simulink model "Blood_Platelet_Count_V2"  (R2022a)
settings: Solver=VariableStepAuto  StartTime=0.0  StopTime=10.0  RelTol=1e-3
model workspace (MAT data in the model file):
  Var = 0
settings Model: Creator=KVJ RAMAN  LastModifiedBy=KVJ RAMAN

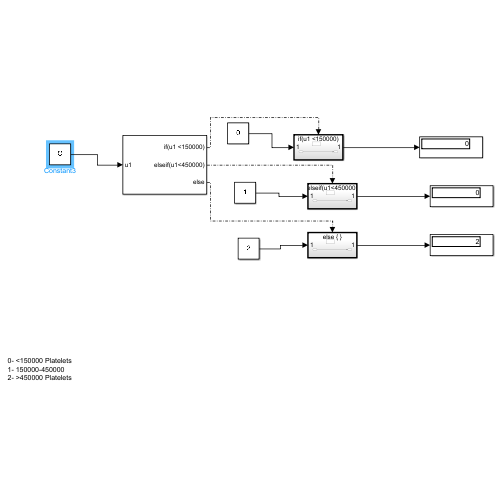
[thumbnail: Simulink's stored preview of the top-level diagram]
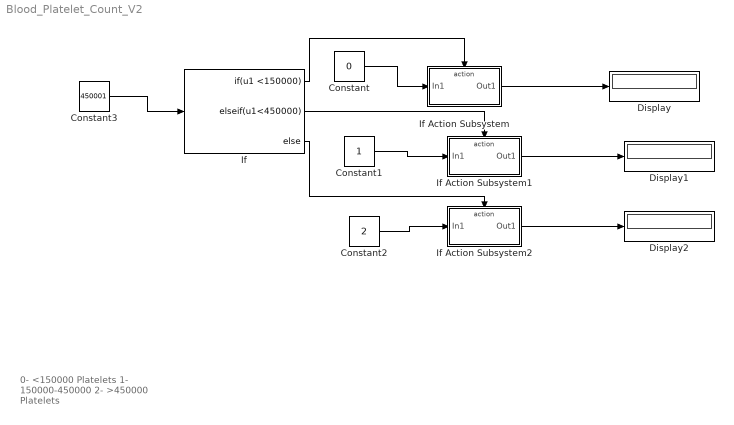
== system Blood_Platelet_Count_V2 ==
  note: 0- <150000 Platelets
      | 1- 150000-450000
      | 2- >450000 Platelets
  Constant : Constant  Value=0
  Constant1 : Constant
  Constant2 : Constant  Value=2
  Constant3 : Constant  Value=450001
  Display : Display
  Display1 : Display
  Display2 : Display
  If : If  IfExpression=u1 <150000  ElseIfExpressions=u1<450000
  If Action Subsystem : Subsystem  TreatAsAtomicUnit=on
  If Action Subsystem1 : Subsystem  TreatAsAtomicUnit=on
  If Action Subsystem2 : Subsystem  TreatAsAtomicUnit=on
  wires:
  If/1 -> If Action Subsystem/Action
  Constant/1 -> If Action Subsystem/1(In1)
  If/2 -> If Action Subsystem1/Action
  If/3 -> If Action Subsystem2/Action
  Constant1/1 -> If Action Subsystem1/1(In1)
  Constant2/1 -> If Action Subsystem2/1(In1)
  If Action Subsystem/1(Out1) -> Display/1
  If Action Subsystem1/1(Out1) -> Display1/1
  If Action Subsystem2/1(Out1) -> Display2/1
  Constant3/1 -> If/1

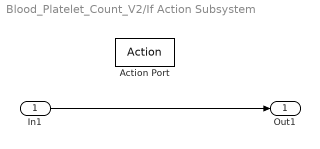
== system Blood_Platelet_Count_V2/If Action Subsystem ==
  In1 : Inport
  Action Port : ActionPort  ActionPortLabel=if(u1 <150000)
  Out1 : Outport
  wires:
  In1/1 -> Out1/1

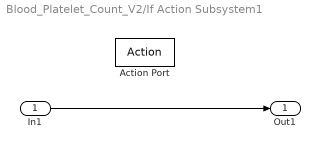
== system Blood_Platelet_Count_V2/If Action Subsystem1 ==
  In1 : Inport
  Action Port : ActionPort  ActionPortLabel=elseif(u1<450000)
  Out1 : Outport
  wires:
  In1/1 -> Out1/1

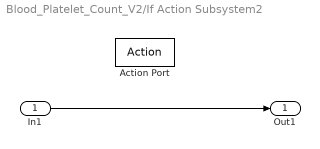
== system Blood_Platelet_Count_V2/If Action Subsystem2 ==
  In1 : Inport
  Action Port : ActionPort  ActionPortLabel=else
  Out1 : Outport
  wires:
  In1/1 -> Out1/1
